simulink model "tank_twin"  (R2021a)
settings: Solver=VariableStepAuto  StartTime=0.0  StopTime=100  RelTol=1e-3
libraries: simulink x2, instrumentlib x1
settings Model: Creator=user  LastModifiedBy=user

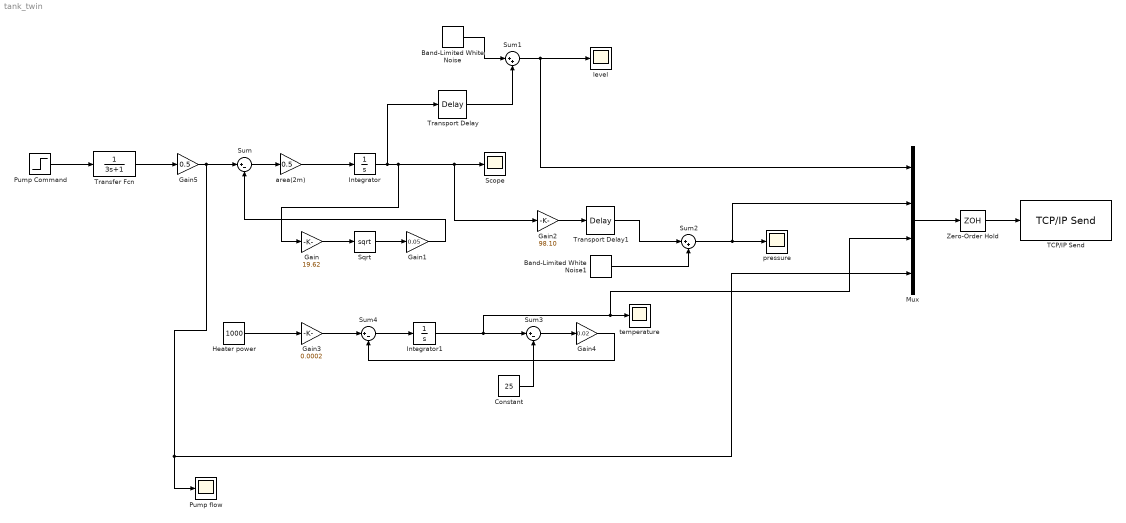
== system tank_twin ==
  Band-Limited White Noise : simulink/Sources/Band-Limited White Noise  Cov=[0.000000000000001]  Ts=0.1  seed=0
  Band-Limited White Noise1 : simulink/Sources/Band-Limited White Noise  Cov=[0.0000001]  Ts=0.1  seed=0
  Constant : Constant  Value=25
  Gain : Gain  Gain=19.62
  Gain1 : Gain  Gain=0.05
  Gain2 : Gain  Gain=98.10
  Gain3 : Gain  Gain=0.0002
  Gain4 : Gain  Gain=0.02
  Gain5 : Gain  Gain=0.5
  Heater power : Constant  Description=Qin  Value=1000
  Integrator : Integrator  LimitOutput=on  UpperSaturationLimit=1000  LowerSaturationLimit=0
  Integrator1 : Integrator  LimitOutput=on  UpperSaturationLimit=200  LowerSaturationLimit=0
  Mux : Mux
  Pump Command : Step  Time=5  SampleTime=0
  Pump flow : Scope
  Scope : Scope
  Sqrt : Sqrt  SaturateOnIntegerOverflow=on
  Sum : Sum  Inputs=|+-
  Sum1 : Sum  Inputs=|++
  Sum2 : Sum  Inputs=|++
  Sum3 : Sum  Inputs=|+-
  Sum4 : Sum  Inputs=|+-
  TCP/IP Send : instrumentlib/TCP//IP Send  Host=127.0.0.1  Port=5005  EnableBlockingMode=on  Timeout=10  ByteOrder=LittleEndian  TransferDelay=on
  Transfer Fcn : TransferFcn  Denominator=[3 1]
  Transport Delay : TransportDelay  DelayTime=0.5
  Transport Delay1 : TransportDelay  DelayTime=0.2
  Zero-Order Hold : ZeroOrderHold  SampleTime=5
  area(2m) : Gain  Gain=0.5
  level : Scope
  pressure : Scope
  temperature : Scope
  wires:
  Sum/1 -> area(2m)/1
  area(2m)/1 -> Integrator/1
  Integrator/1 -> Transport Delay/1, Gain/1, Gain2/1, Scope/1
  Gain/1 -> Sqrt/1
  Sqrt/1 -> Gain1/1
  Gain1/1 -> Sum/2
  Band-Limited White Noise/1 -> Sum1/1
  Transport Delay/1 -> Sum1/2
  Gain2/1 -> Transport Delay1/1
  Transport Delay1/1 -> Sum2/1
  Band-Limited White Noise1/1 -> Sum2/2
  Heater power/1 -> Gain3/1
  Constant/1 -> Sum3/2
  Sum3/1 -> Gain4/1
  Gain3/1 -> Sum4/1
  Sum4/1 -> Integrator1/1
  Gain4/1 -> Sum4/2
  Transfer Fcn/1 -> Gain5/1
  Pump Command/1 -> Transfer Fcn/1
  Zero-Order Hold/1 -> TCP/IP Send/1
  Mux/1 -> Zero-Order Hold/1
  Sum1/1 -> Mux/1, level/1
  Sum2/1 -> Mux/2, pressure/1
  Integrator1/1 -> Mux/3, temperature/1, Sum3/1
  Gain5/1 -> Mux/4, Pump flow/1, Sum/1
